simulink model "Original"  (Simulink 7.5)
settings: Solver=ode45  StartTime=0.0  StopTime=5000  RelTol=1e-3
values from neighbouring files (symbols this model uses):
  fmax = Ki/2    (= 0.5)    [Original1.m]
undefined symbols (not defined in the file or in its folder): D, I, lb, ub, xi
libraries: fuzblock x1, powerlib x1
settings Model: Creator=Suji Kumar  LastModifiedBy=Suji Kumar

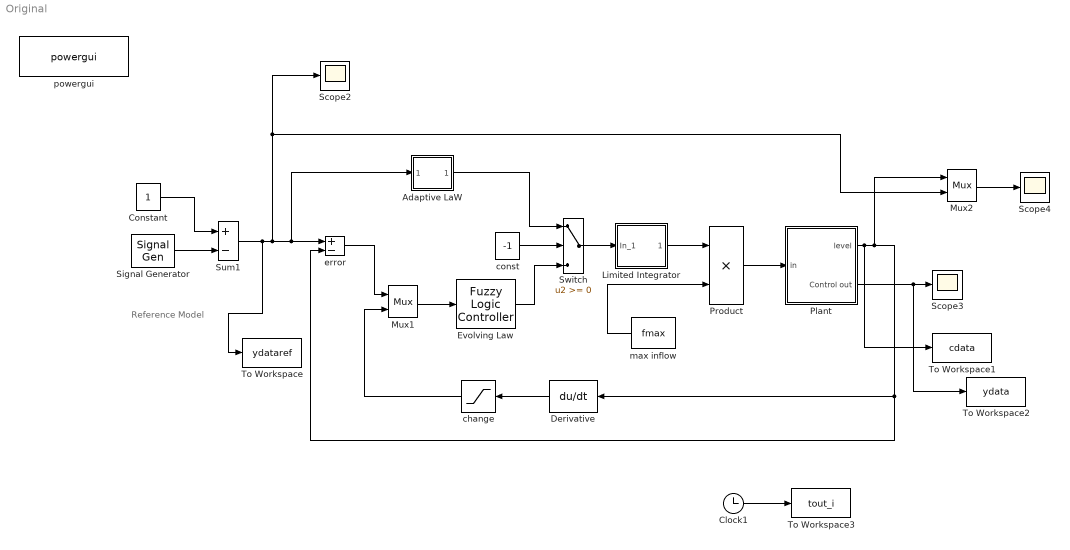
== system Original ==
  note: Reference Model
  Adaptive LaW : Subsystem  mask(PID Controller){P=20,  I=0.5,  D=0.5}
      mask prompts: P "Proportional:";  I "Integral";  D "Derivative:"
      mask help:
      | Enter expressions for proportional, integral, and derivative terms.
      | P+I/s+Ds
      mask Help: This block implements a PID controller where parameters are entered for the Proportional, Integral and Derivative terms. Unmask this block to see how it works. The derivative term is implemented using a true derivative block.
      mask Display: disp('PID')
  Clock1 : Clock
      settings: Decimation=10
  Constant : Constant  OutDataType=sfix(16)  OutScaling=2^0
  Derivative : Derivative
  Evolving Law : fuzblock/Fuzzy Logic  Controller  SystemSampleTime=-1  fis=rule_data
  Limited Integrator : Subsystem  mask(Limited integrator.){lb =0,  ub =1,  xi =0}
      mask prompts: lb  "Lower bound:";  ub  "Upper bound:";  xi  "Initial condition"
      mask help: Limited integrator
      mask Help: Implements a limited integrator with \nan expression of the form:\n\nif(x<=lb and u<0) or (x>=ub and u>0)\n\txdot=0\nelse\n\txdot=u.
      mask Display: plot(-1,-0.2,3.5,1.2,[0.05,1,2,2.9],[0,0,1,1]);disp(' 1/s    ')
  Mux1 : Mux  Inputs=2
  Mux2 : Mux  Inputs=2
  Plant : Subsystem
  Product : Product  OutDataType=sfix(16)  OutScaling=2^0  SaturateOnIntegerOverflow=on  RndMeth=Zero  InputSameDT=on  OutDataTypeStr=Inherit: Same as first input
  Scope2 : Scope
      settings: TickLabels=on  TimeRange=200  YMin=0.8  YMax=1.2  SaveName=ScopeData2  DataFormat=Array
  Scope3 : Scope
      settings: TickLabels=on  TimeRange=200  YMin=0.15  YMax=0.28  SaveName=ScopeData3  DataFormat=Array
  Scope4 : Scope
      settings: TickLabels=on  TimeRange=200  YMin=0.45  YMax=1.5  DataFormat=Array
  Signal Generator : SignalGenerator  WaveForm=square  Amplitude=0.500000  Frequency=0.100000  Units=rad/sec
  Sum1 : Sum  Inputs=+-  OutDataType=sfix(16)  OutScaling=2^0  SaturateOnIntegerOverflow=on  InputSameDT=on  OutDataTypeStr=Inherit: Same as first input
  Switch : Switch  SaturateOnIntegerOverflow=on  InputSameDT=on
  To Workspace : ToWorkspace  VariableName=ydataref  SampleTime=-1  SaveFormat=Structure
  To Workspace1 : ToWorkspace  VariableName=cdata  SampleTime=-1  SaveFormat=Structure
  To Workspace2 : ToWorkspace  VariableName=ydata  SampleTime=-1  SaveFormat=Structure
  To Workspace3 : ToWorkspace  VariableName=tout_i  SampleTime=-1  SaveFormat=Array
  change : Saturate  UpperLimit=0.1  LowerLimit=-0.1
  const : Constant  Value=-1  OutDataType=sfix(16)  OutScaling=2^0
  error : Sum  Inputs=+-  OutDataType=sfix(16)  OutScaling=2^0  SaturateOnIntegerOverflow=on  InputSameDT=on  OutDataTypeStr=Inherit: Same as first input
  max inflow : Constant  Value=fmax  OutDataType=sfix(16)  OutScaling=2^0
  powergui : powerlib/powergui  Priority=1  SystemSampleTime=-1  SimulationMode=Discrete  SampleTime=4e-5  frequency=60  SPID=off  DisableSnubberDevices=off  DisableRonSwitches=off  DisableVfSwitches=off  SwTol=0  Interpol=off  frequencyindice=0  echomessages=off  HookPort=off  DisplayEquations=off  FunctionMessages=off  EnableUseOfTLC=off  x0status=blocks  RestoreLinks=warning  ResistiveCurrentMeasurement=off  Frange=[0:2:500]  Ylog=off  Xlog=on  ShowGrid=off  save=off  variable=ZData  ZoomFFT=on  StartTime=0.0  cycles=1  DisplayStyle=1  fundamental=60  FreqAxis=off  MaxFrequency=1000  frequencyindicesteady=1  RmsSteady=1  display=off  Ts=0  methode=off
  wires:
  Sum1/1 -> Mux2/2, Scope2/1, error/1, Adaptive LaW/1(In_1), To Workspace/1
  error/1 -> Mux1/1
  Mux1/1 -> Evolving Law/1
  Evolving Law/1 -> Switch/3
  const/1 -> Switch/2
  Adaptive LaW/1(Out_1) -> Switch/1
  Switch/1 -> Limited Integrator/1(In_1)
  Limited Integrator/1(Out_1) -> Product/1
  max inflow/1 -> Product/2
  Product/1 -> Plant/1(in)
  Plant/1(level) -> Mux2/1, error/2, Derivative/1, To Workspace1/1
  Derivative/1 -> change/1
  change/1 -> Mux1/2
  Mux2/1 -> Scope4/1
  Constant/1 -> Sum1/1
  Signal Generator/1 -> Sum1/2
  Plant/2(Control out) -> Scope3/1, To Workspace2/1
  Clock1/1 -> To Workspace3/1

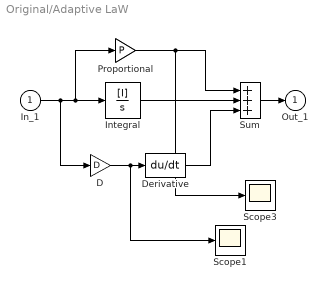
== system Original/Adaptive LaW ==
  In_1 : Inport  OutDataType=sfix(16)  OutScaling=2^0
  D : Gain  Gain=D  ParameterDataType=sfix(16)  ParameterScaling=2^0  OutDataType=sfix(16)  OutScaling=2^0  SaturateOnIntegerOverflow=on  OutDataTypeStr=Inherit: Same as input  ParamDataTypeStr=Inherit: Same as input
  Derivative : Derivative
  Integral : TransferFcn  Numerator=[I]  Denominator=[1 0]
  Proportional : Gain  Gain=P  ParameterDataType=sfix(16)  ParameterScaling=2^0  OutDataType=sfix(16)  OutScaling=2^0  SaturateOnIntegerOverflow=on  OutDataTypeStr=Inherit: Same as input  ParamDataTypeStr=Inherit: Same as input
  Scope1 : Scope
      settings: TickLabels=on  TimeRange=200  YMin=-0.5  YMax=0.55  SaveName=ScopeData4  DataFormat=Array
  Scope3 : Scope
      settings: TickLabels=on  TimeRange=200  YMin=4.6  YMax=6.5  DataFormat=Array
  Sum : Sum  Inputs=+++  OutDataType=sfix(16)  OutScaling=2^0  SaturateOnIntegerOverflow=on  InputSameDT=on  OutDataTypeStr=Inherit: Same as first input
  Out_1 : Outport  OutDataType=sfix(16)  OutScaling=2^0  InitialOutput=0
  wires:
  Proportional/1 -> Sum/1, Scope3/1
  Integral/1 -> Sum/2
  Derivative/1 -> Sum/3
  In_1/1 -> Integral/1, Proportional/1, D/1
  Sum/1 -> Out_1/1
  D/1 -> Derivative/1, Scope1/1

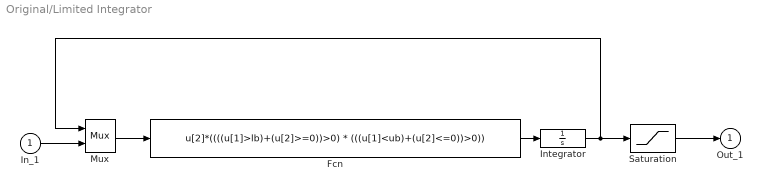
== system Original/Limited Integrator ==
  In_1 : Inport  OutDataType=sfix(16)  OutScaling=2^0
  Fcn : Fcn  Expr=u[2]*((((u[1]>lb)+(u[2]>=0))>0) * (((u[1]<ub)+(u[2]<=0))>0))
  Integrator : Integrator  InitialCondition=xi
  Mux : Mux  Inputs=2
  Saturation : Saturate  UpperLimit=ub  LowerLimit=lb
  Out_1 : Outport  OutDataType=sfix(16)  OutScaling=2^0  InitialOutput=0
  wires:
  Integrator/1 -> Saturation/1, Mux/1
  Fcn/1 -> Integrator/1
  Mux/1 -> Fcn/1
  In_1/1 -> Mux/2
  Saturation/1 -> Out_1/1

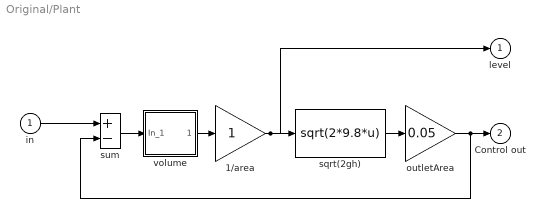
== system Original/Plant ==
  in : Inport  OutDataType=sfix(16)  OutScaling=2^0
  1/area : Gain  ParameterDataType=sfix(16)  ParameterScaling=2^0  OutDataType=sfix(16)  OutScaling=2^0  SaturateOnIntegerOverflow=on  OutDataTypeStr=Inherit: Same as input  ParamDataTypeStr=Inherit: Same as input
  outletArea : Gain  Gain=0.05  ParameterDataType=sfix(16)  ParameterScaling=2^0  OutDataType=sfix(16)  OutScaling=2^0  SaturateOnIntegerOverflow=on  OutDataTypeStr=Inherit: Same as input  ParamDataTypeStr=Inherit: Same as input
  sqrt(2gh) : Fcn  Expr=sqrt(2*9.8*u)
  sum : Sum  Inputs=+-  OutDataType=sfix(16)  OutScaling=2^0  SaturateOnIntegerOverflow=on  InputSameDT=on  OutDataTypeStr=Inherit: Same as first input
  volume : Subsystem  mask(Limited integrator.){lb =0,  ub =2,  xi =0.5}
      mask prompts: lb  "Lower bound:";  ub  "Upper bound:";  xi  "Initial condition"
      mask help: Limited integrator
      mask Help: Implements a limited integrator with \nan expression of the form:\n\nif(x<=lb and u<0) or (x>=ub and u>0)\n\txdot=0\nelse\n\txdot=u.
      mask Display: plot(-1,-0.2,3.5,1.2,[0.05,1,2,2.9],[0,0,1,1]);disp(' 1/s    ')
  level : Outport  OutDataType=sfix(16)  OutScaling=2^0  InitialOutput=0
  Control out : Outport  Port=2  OutDataType=sfix(16)  OutScaling=2^0  InitialOutput=0
  wires:
  outletArea/1 -> Control out/1, sum/2
  sqrt(2gh)/1 -> outletArea/1
  1/area/1 -> sqrt(2gh)/1, level/1
  volume/1(Out_1) -> 1/area/1
  in/1 -> sum/1
  sum/1 -> volume/1(In_1)

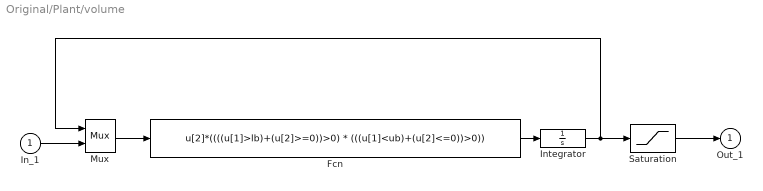
== system Original/Plant/volume ==
  In_1 : Inport  OutDataType=sfix(16)  OutScaling=2^0
  Fcn : Fcn  Expr=u[2]*((((u[1]>lb)+(u[2]>=0))>0) * (((u[1]<ub)+(u[2]<=0))>0))
  Integrator : Integrator  InitialCondition=xi
  Mux : Mux  Inputs=2
  Saturation : Saturate  UpperLimit=ub  LowerLimit=lb
  Out_1 : Outport  OutDataType=sfix(16)  OutScaling=2^0  InitialOutput=0
  wires:
  Integrator/1 -> Saturation/1, Mux/1
  Fcn/1 -> Integrator/1
  Mux/1 -> Fcn/1
  In_1/1 -> Mux/2
  Saturation/1 -> Out_1/1
